simulink model "AutonomousDriving"  (R2026b)
settings: Solver=FixedStepDiscrete  StopTime=25  FixedStep=0.1
undefined symbols (not defined in the file or in its folder): sih
settings Model: Creator=Hp  LastModifiedBy=Hp

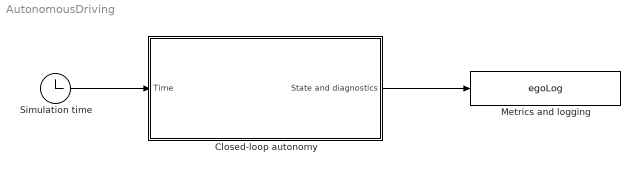
== system AutonomousDriving ==
  Closed-loop autonomy : Subsystem
  Metrics and logging : ToWorkspace  VariableName=egoLog  SaveFormat=Timeseries  SampleTime=-1
  Simulation time : Clock
  wires:
  Simulation time/1 -> Closed-loop autonomy/1(Time)
  Closed-loop autonomy/1(State and diagnostics) -> Metrics and logging/1

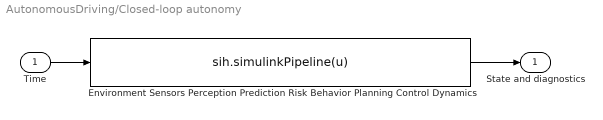
== system AutonomousDriving/Closed-loop autonomy ==
  Time : Inport
  Environment Sensors Perception Prediction Risk Behavior Planning Control Dynamics : MATLABFcn  MATLABFcn=sih.simulinkPipeline(u)  OutputDimensions=10  SampleTime=0.1
  State and diagnostics : Outport
  wires:
  Time/1 -> Environment Sensors Perception Prediction Risk Behavior Planning Control Dynamics/1
  Environment Sensors Perception Prediction Risk Behavior Planning Control Dynamics/1 -> State and diagnostics/1
